simulink model "Automatisierung_subsystem_test"  (R2016b)
settings: Solver=VariableStepAuto  StartTime=0.0  StopTime=300.0  RelTol=1e-3
model workspace (MAT data in the model file):
  a = Simulink.Parameter
  a.DataType = 'auto'
  a.Dimensions = [0 0]
  b = Simulink.Parameter
  b.DataType = 'auto'
  b.Dimensions = [0 0]
settings Model: Creator=Fritz  LastModifiedBy=Fritz

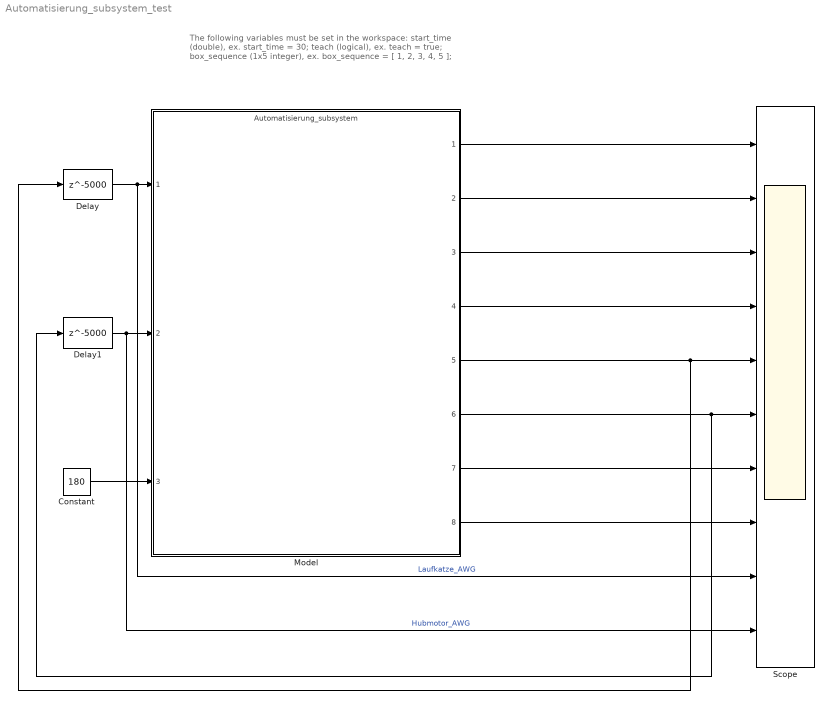
== system Automatisierung_subsystem_test ==
  note: The following variables must be set in the workspace:
      | start_time (double), ex. start_time = 30;
      | teach (logical), ex. teach = true;
      | box_sequence (1x5 integer), ex. box_sequence = [ 1, 2, 3, 4, 5 ];
  Constant : Constant  Value=180
  Delay : Delay  DelayLength=5000
  Delay1 : Delay  DelayLength=5000
  Model : ModelReference  ModelNameDialog=Automatisierung_subsystem.slx  SimulationMode=Normal  ModelReferenceVersion=1.72
  Scope : Scope  NumInputPorts=10
  wires:
  Model/1 -> Scope/1
  Model/2 -> Scope/2
  Model/3 -> Scope/3
  Model/4 -> Scope/4
  Model/5 -> Delay/1, Scope/5
  Model/7 -> Scope/7
  Model/8 -> Scope/8
  Delay/1 -> Scope/9, Model/1  "Laufkatze_AWG"
  Delay1/1 -> Scope/10, Model/2  "Hubmotor_AWG"
  Constant/1 -> Model/3
  Model/6 -> Delay1/1, Scope/6
